simulink model "uav"  (R2024b)
settings: Solver=VariableStepAuto  StartTime=0.0  StopTime=30  RelTol=1e-3
libraries: slpidlib x3, shared6dof x1, aerolibadyn x1, aerolibanimutils x1
settings Model: Creator=91964  LastModifiedBy=91964

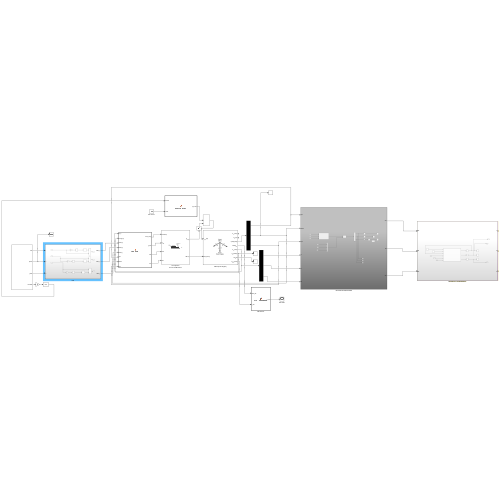
[thumbnail: Simulink's stored preview of the top-level diagram]
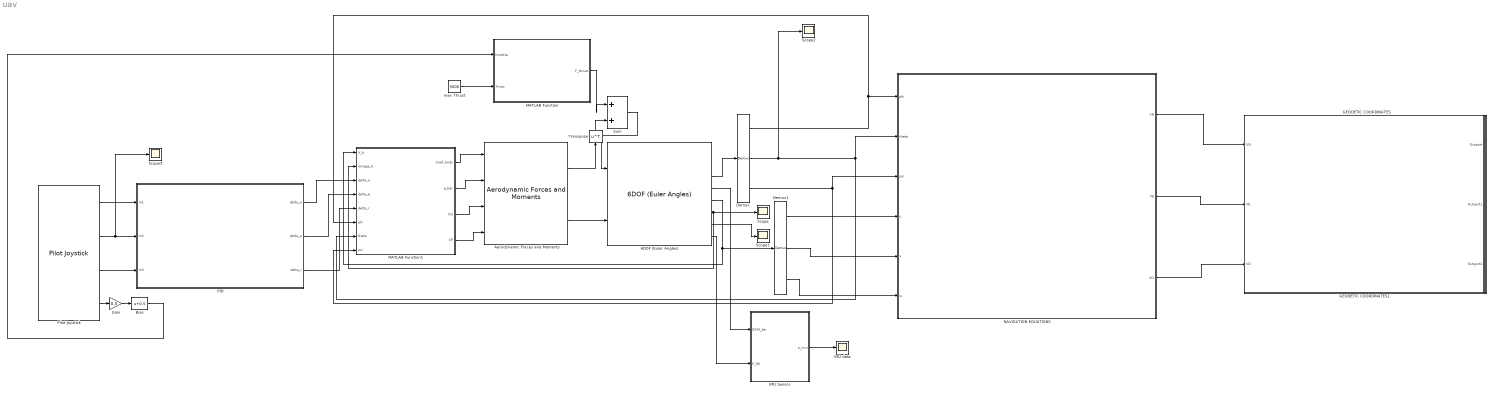
== system uav ==
  6DOF (Euler Angles) : shared6dof/6DOF (Euler Angles)  units=Metric (MKS)  mtype=Fixed  rep=Euler Angles  xme_0=[0 0 100]  Vm_0=[30 0 0]  eul_0=[0 0 0]  pm_0=[0 0 0]  mass_0=60  mass_e=0.5  mass_f=2.0  inertia=eye(3)  inertia_e=eye(3)  inertia_f=2*eye(3)  k_quat=1.0  vre_flag=on  abi_flag=off  aMode=0  xme_statename=''  Vm_statename=''  eul_statename=''  quat_statename=''  pm_statename=''  mass_statename=''
  "Aerodynamic Forces and Moments " : aerolibadyn/Aerodynamic Forces and Moments   inputAxes=Body  outputForceAxes=Body  outputMomentAxes=Body  S=1  b=1  cbar=1
  Bias : Bias  Bias=0.5  SaturateOnIntegerOverflow=off
  Demux : Demux  Outputs=3
  Demux1 : Demux  Outputs=3
  GEODETIC COORDINATES : Subsystem
  GEODETIC COORDINATES1 : Subsystem
  Gain : Gain  Gain=0.5
  IMU Sensor : MATLAB Function  TreatAsAtomicUnit=on
  IMU data : Scope
  MATLAB Function : MATLAB Function  TreatAsAtomicUnit=on
  MATLAB Function1 : MATLAB Function  TreatAsAtomicUnit=on
  NAVIGATION EQUATIONS : Subsystem
  PID : Subsystem
  Pilot Joystick : aerolibanimutils/Pilot Joystick  JoystickID=Joystick1  OutputConfiguration=FourAxis  SampleTime=1/30
  Scope{,1..3} (4 alike) : Scope
  Sum : Sum  Inputs=|++
  Transpose : Math  Operator=transpose
  "max Thrust " : Constant  Value=5000
  wires:
  "Aerodynamic Forces and Moments "/1 -> Transpose/1
  "Aerodynamic Forces and Moments "/2 -> 6DOF (Euler Angles)/2
  NAVIGATION EQUATIONS/2(VE) -> GEODETIC COORDINATES/2(VE)
  NAVIGATION EQUATIONS/1(VN) -> GEODETIC COORDINATES/1(VN)
  NAVIGATION EQUATIONS/3(VD) -> GEODETIC COORDINATES/3(VD)
  Demux/2 -> MATLAB Function1/7(theta), NAVIGATION EQUATIONS/2(theta), Scope2/1
  6DOF (Euler Angles)/3 -> Demux/1
  Demux/3 -> MATLAB Function1/8(psi), NAVIGATION EQUATIONS/3(psi)
  6DOF (Euler Angles)/5 -> MATLAB Function1/1(V_b), Demux1/1
  Demux1/1 -> NAVIGATION EQUATIONS/4(u)
  Demux1/2 -> NAVIGATION EQUATIONS/5(v)
  Demux1/3 -> NAVIGATION EQUATIONS/6(w)
  Pilot Joystick/1 -> PID/1(In1)
  Pilot Joystick/2 -> Scope3/1, PID/2(In2)
  Pilot Joystick/3 -> PID/3(In3)
  PID/1(delta_a) -> MATLAB Function1/3(delta_a)
  PID/2(delta_e) -> MATLAB Function1/4(delta_e)
  PID/3(delta_r) -> MATLAB Function1/5(delta_r)
  6DOF (Euler Angles)/4 -> IMU Sensor/1(DCM_be)
  6DOF (Euler Angles)/8 -> IMU Sensor/2(A_bb)
  IMU Sensor/1(a_imu) -> IMU data/1
  6DOF (Euler Angles)/6 -> MATLAB Function1/2(omega_b), Scope/1
  6DOF (Euler Angles)/7 -> Scope1/1
  Pilot Joystick/4 -> Gain/1
  "max Thrust "/1 -> MATLAB Function/2(Tmax)
  Gain/1 -> Bias/1
  Bias/1 -> MATLAB Function/1(throttle)
  MATLAB Function/1(F_thrust) -> Sum/1
  Sum/1 -> 6DOF (Euler Angles)/1
  Transpose/1 -> Sum/2
  Demux/1 -> MATLAB Function1/6(phi), NAVIGATION EQUATIONS/1(phi)
  MATLAB Function1/1(Coef_body) -> "Aerodynamic Forces and Moments "/1
  MATLAB Function1/2(q_bar) -> "Aerodynamic Forces and Moments "/2
  MATLAB Function1/3(CG) -> "Aerodynamic Forces and Moments "/3
  MATLAB Function1/4(CP) -> "Aerodynamic Forces and Moments "/4

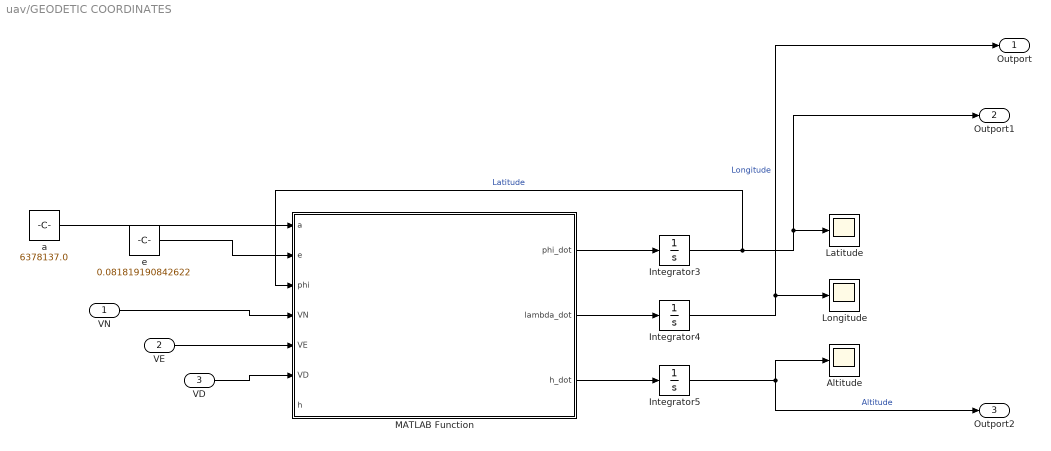
== system uav/GEODETIC COORDINATES ==
  VN : Inport
  VE : Inport  Port=2
  VD : Inport  Port=3
  Altitude : Scope
  Integrator3 : Integrator
  Integrator4 : Integrator
  Integrator5 : Integrator
  Latitude : Scope
  Longitude : Scope
  MATLAB Function : MATLAB Function  TreatAsAtomicUnit=on
  a : Constant  Value=6378137.0
  e : Constant  Value=0.081819190842622
  Outport : Outport
  Outport1 : Outport  Port=2
  Outport2 : Outport  Port=3
  wires:
  MATLAB Function/3(h_dot) -> Integrator5/1
  e/1 -> MATLAB Function/2(e)
  MATLAB Function/2(lambda_dot) -> Integrator4/1
  MATLAB Function/1(phi_dot) -> Integrator3/1
  a/1 -> MATLAB Function/1(a)
  Integrator4/1 -> Outport/1, Longitude/1  "Longitude"
  Integrator3/1 -> MATLAB Function/3(phi), Outport1/1, Latitude/1  "Latitude"
  Integrator5/1 -> Altitude/1, Outport2/1  "Altitude"
  VN/1 -> MATLAB Function/4(VN)
  VD/1 -> MATLAB Function/6(VD)
  VE/1 -> MATLAB Function/5(VE)

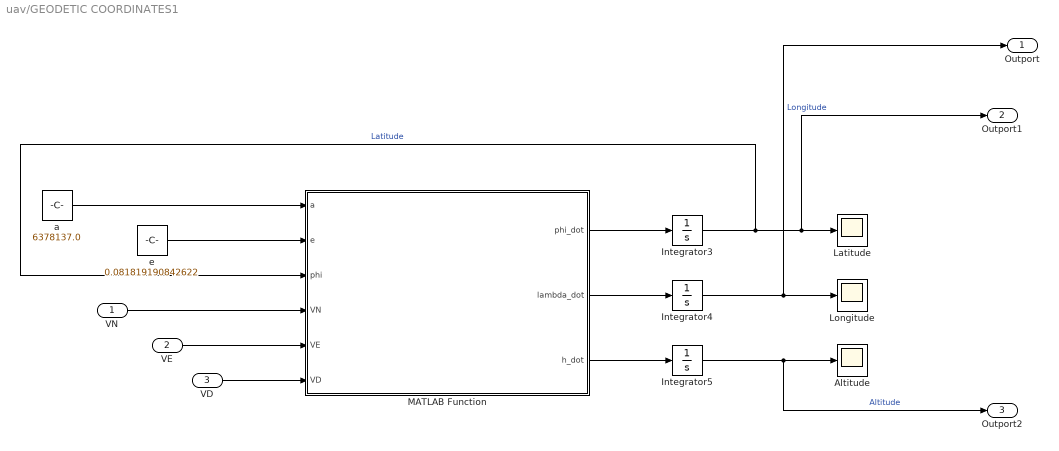
== system uav/GEODETIC COORDINATES1 ==
  VN : Inport
  VE : Inport  Port=2
  VD : Inport  Port=3
  Altitude : Scope
  Integrator3 : Integrator
  Integrator4 : Integrator
  Integrator5 : Integrator
  Latitude : Scope
  Longitude : Scope
  MATLAB Function : MATLAB Function  TreatAsAtomicUnit=on
  a : Constant  Value=6378137.0
  e : Constant  Value=0.081819190842622
  Outport : Outport
  Outport1 : Outport  Port=2
  Outport2 : Outport  Port=3
  wires:
  VE/1 -> MATLAB Function/5(VE)
  VD/1 -> MATLAB Function/6(VD)
  VN/1 -> MATLAB Function/4(VN)
  Integrator5/1 -> Altitude/1, Outport2/1  "Altitude"
  Integrator3/1 -> Latitude/1, Outport1/1, MATLAB Function/3(phi)  "Latitude"
  Integrator4/1 -> Longitude/1, Outport/1  "Longitude"
  a/1 -> MATLAB Function/1(a)
  MATLAB Function/1(phi_dot) -> Integrator3/1
  MATLAB Function/2(lambda_dot) -> Integrator4/1
  e/1 -> MATLAB Function/2(e)
  MATLAB Function/3(h_dot) -> Integrator5/1

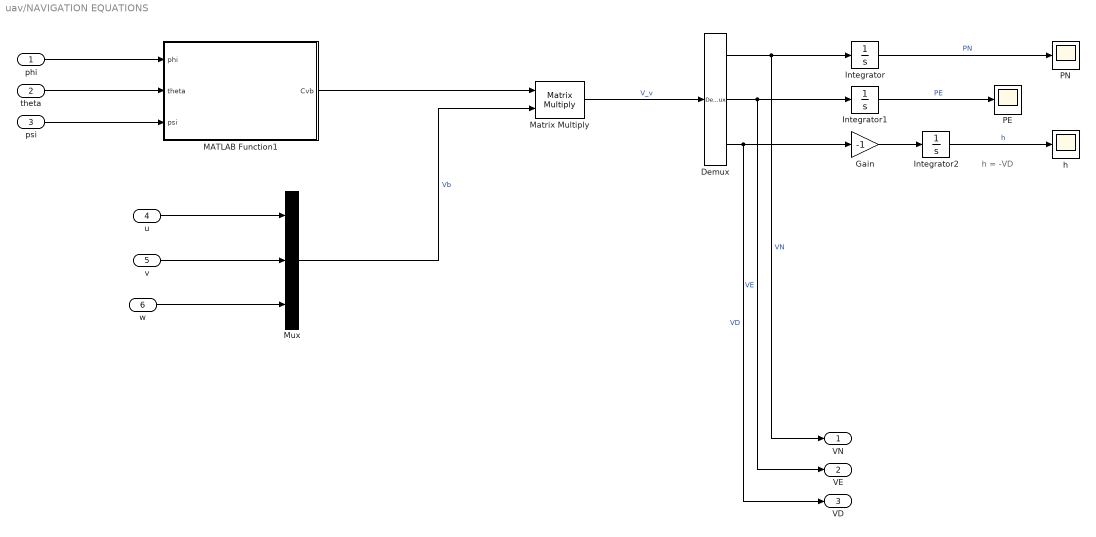
== system uav/NAVIGATION EQUATIONS ==
  note: h = -VD
  phi : Inport
  theta : Inport  Port=2
  psi : Inport  Port=3
  u : Inport  Port=4
  v : Inport  Port=5
  w : Inport  Port=6
  Demux : Demux  Outputs=3
  Gain : Gain  Gain=-1
  Integrator : Integrator
  Integrator1 : Integrator
  Integrator2 : Integrator
  MATLAB Function1 : MATLAB Function  TreatAsAtomicUnit=on
  Matrix Multiply : Product  Multiplication=Matrix(*)
  Mux : Mux  Inputs=3
  PE : Scope
  PN : Scope
  h : Scope
  VN : Outport
  VE : Outport  Port=2
  VD : Outport  Port=3
  wires:
  Demux/1 -> VN/1, Integrator/1  "VN"
  Gain/1 -> Integrator2/1
  Demux/2 -> VE/1, Integrator1/1  "VE"
  Mux/1 -> Matrix Multiply/2  "Vb"
  MATLAB Function1/1(Cvb) -> Matrix Multiply/1
  Demux/3 -> VD/1, Gain/1  "VD"
  v/1 -> Mux/2
  Integrator/1 -> PN/1  "PN"
  Matrix Multiply/1 -> Demux/1  "V_v"
  Integrator1/1 -> PE/1  "PE"
  Integrator2/1 -> h/1  "h"
  theta/1 -> MATLAB Function1/2(theta)
  psi/1 -> MATLAB Function1/3(psi)
  w/1 -> Mux/3
  u/1 -> Mux/1
  phi/1 -> MATLAB Function1/1(phi)

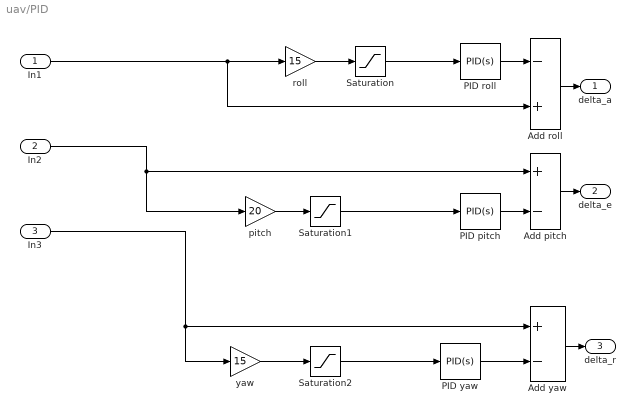
== system uav/PID ==
  In1 : Inport
  In2 : Inport  Port=2
  In3 : Inport  Port=3
  Add pitch : Sum  Inputs=+-
  Add roll : Sum  Inputs=-+
  Add yaw : Sum  Inputs=+-
  PID pitch : slpidlib/PID Controller  Controller=PID  Form=Parallel  TimeDomain=Continuous-time  UseExternalTs=off  SampleTime=-1  IntegratorMethod=Forward Euler  FilterMethod=Forward Euler  ControllerParametersSource=internal  P=1  I=1  UseKiTs=off  D=0  UseExternalDerivativeSource=off  N=100  UseFilter=on  TunerSelectOption=Transfer Function Based (PID Tuner App)  InitialConditionSource=internal  InitialConditionForIntegrator=0  InitialConditionForFilter=0  DifferentiatorICPrevScaledInput=0  ExternalReset=none  TrackingMode=off  Kt=1  LimitOutput=off  SatLimitsSource=internal  UpperSaturationLimit=inf  LowerSaturationLimit=-inf  LinearizeAsGain=on  AntiWindupMode=none  Kb=1  LimitIntegrator=off  UpperIntegratorSaturationLimit=inf  LowerIntegratorSaturationLimit=-inf  POutMin=[]  POutMax=[]  IOutMin=[]  IOutMax=[]  DOutMin=[]  DOutMax=[]  NOutMin=[]  NOutMax=[]  SumOutMin=[]  SumOutMax=[]  SaturationOutMin=[]  SaturationOutMax=[]  PParamMin=[]  PParamMax=[]  IParamMin=[]  IParamMax=[]  DParamMin=[]  DParamMax=[]  NParamMin=[]  NParamMax=[]  KbParamMin=[]  KbParamMax=[]  KtParamMin=[]  KtParamMax=[]  KbOutMin=[]  KbOutMax=[]  KtOutMin=[]  KtOutMax=[]  IntegratorOutMin=[]  IntegratorOutMax=[]  FilterOutMin=[]  FilterOutMax=[]  SumI1OutMin=[]  SumI1OutMax=[]  SumI2OutMin=[]  SumI2OutMax=[]  SumI3OutMin=[]  SumI3OutMax=[]  SumI4OutMin=[]  SumI4OutMax=[]  SumDOutMin=[]  SumDOutMax=[]  DifferentiatorOutMin=[]  DifferentiatorOutMax=[]  FilterDiffOutCoefMin=[]  FilterDiffOutCoefMax=[]  ReciprocalOutMin=[]  ReciprocalOutMax=[]  SumDenOutMin=[]  SumDenOutMax=[]  SumNumOutMin=[]  SumNumOutMax=[]  DivideOutMin=[]  DivideOutMax=[]  UdiffTsProdOutMin=[]  UdiffTsProdOutMax=[]  NTsProdOutMin=[]  NTsProdOutMax=[]  UintegralTsProdOutMin=[]  UintegralTsProdOutMax=[]  UngainTsProdOutMin=[]  UngainTsProdOutMax=[]  ClampingZeroOutDataTypeStr=Inherit: Inherit via back propagation  ClampingZeroOutMin=[]  ClampingZeroOutMax=[]  FilterDenConstantOutDataTypeStr=Inherit: Inherit via back propagation  FilterDenConstantOutMin=[]  FilterDenConstantOutMax=[]  PCopyOutDataTypeStr=Inherit: Inherit via back propagation  PCopyOutMin=[]  PCopyOutMax=[]  NCopyOutDataTypeStr=Inherit: Inherit via back propagation  NCopyOutMin=[]  NCopyOutMax=[]  IntegratorContinuousStateAttributes=''  IntegratorStateMustResolveToSignalObject=off  IntegratorRTWStateStorageClass=Auto  FilterContinuousStateAttributes=''  FilterStateMustResolveToSignalObject=off  FilterRTWStateStorageClass=Auto  ParallelPVariant=InternalParameters  IdealPVariant=Disabled  IVariant=InternalParameters  DVariant=InternalParameters  IntegratorVariant=Continuous  SatVariant=Disabled  AWVariant=Passthrough  PCopyVariant=Disabled  TRVariant=Disabled  FdbkBlocksVariant=Forward  IdealPFdbkVariant=Disabled  SatFdbkVariant=Disabled  DerivativeFilterVariant=ContFilter  NVariant=InternalParameters  NCopyVariant=Disabled  FilterICVariant=InternalICsFilter  IntegratorICVariant=InternalICs  ExternalResetVariant=Disabled  TRSumVariant=Passthrough  SumFdbkVariant=Disabled  SumVariant=Sum_PID  TsampFilterVariant=InternalTs  TsampNgainVariant=Passthrough  TsampIntegralVariant=Disabled_SignalSpec  ExternalSaturationOutDataTypeStr=Inherit: Same as second input  DerivativeSourceVariant=ErrorSignal  PreIntVariant=InternalPreInt
  PID roll : slpidlib/PID Controller  Controller=PID  Form=Parallel  TimeDomain=Continuous-time  UseExternalTs=off  SampleTime=-1  IntegratorMethod=Forward Euler  FilterMethod=Forward Euler  ControllerParametersSource=internal  P=1  I=1  UseKiTs=off  D=0  UseExternalDerivativeSource=off  N=100  UseFilter=on  TunerSelectOption=Transfer Function Based (PID Tuner App)  InitialConditionSource=internal  InitialConditionForIntegrator=0  InitialConditionForFilter=0  DifferentiatorICPrevScaledInput=0  ExternalReset=none  TrackingMode=off  Kt=1  LimitOutput=off  SatLimitsSource=internal  UpperSaturationLimit=inf  LowerSaturationLimit=-inf  LinearizeAsGain=on  AntiWindupMode=none  Kb=1  LimitIntegrator=off  UpperIntegratorSaturationLimit=inf  LowerIntegratorSaturationLimit=-inf  POutMin=[]  POutMax=[]  IOutMin=[]  IOutMax=[]  DOutMin=[]  DOutMax=[]  NOutMin=[]  NOutMax=[]  SumOutMin=[]  SumOutMax=[]  SaturationOutMin=[]  SaturationOutMax=[]  PParamMin=[]  PParamMax=[]  IParamMin=[]  IParamMax=[]  DParamMin=[]  DParamMax=[]  NParamMin=[]  NParamMax=[]  KbParamMin=[]  KbParamMax=[]  KtParamMin=[]  KtParamMax=[]  KbOutMin=[]  KbOutMax=[]  KtOutMin=[]  KtOutMax=[]  IntegratorOutMin=[]  IntegratorOutMax=[]  FilterOutMin=[]  FilterOutMax=[]  SumI1OutMin=[]  SumI1OutMax=[]  SumI2OutMin=[]  SumI2OutMax=[]  SumI3OutMin=[]  SumI3OutMax=[]  SumI4OutMin=[]  SumI4OutMax=[]  SumDOutMin=[]  SumDOutMax=[]  DifferentiatorOutMin=[]  DifferentiatorOutMax=[]  FilterDiffOutCoefMin=[]  FilterDiffOutCoefMax=[]  ReciprocalOutMin=[]  ReciprocalOutMax=[]  SumDenOutMin=[]  SumDenOutMax=[]  SumNumOutMin=[]  SumNumOutMax=[]  DivideOutMin=[]  DivideOutMax=[]  UdiffTsProdOutMin=[]  UdiffTsProdOutMax=[]  NTsProdOutMin=[]  NTsProdOutMax=[]  UintegralTsProdOutMin=[]  UintegralTsProdOutMax=[]  UngainTsProdOutMin=[]  UngainTsProdOutMax=[]  ClampingZeroOutDataTypeStr=Inherit: Inherit via back propagation  ClampingZeroOutMin=[]  ClampingZeroOutMax=[]  FilterDenConstantOutDataTypeStr=Inherit: Inherit via back propagation  FilterDenConstantOutMin=[]  FilterDenConstantOutMax=[]  PCopyOutDataTypeStr=Inherit: Inherit via back propagation  PCopyOutMin=[]  PCopyOutMax=[]  NCopyOutDataTypeStr=Inherit: Inherit via back propagation  NCopyOutMin=[]  NCopyOutMax=[]  IntegratorContinuousStateAttributes=''  IntegratorStateMustResolveToSignalObject=off  IntegratorRTWStateStorageClass=Auto  FilterContinuousStateAttributes=''  FilterStateMustResolveToSignalObject=off  FilterRTWStateStorageClass=Auto  ParallelPVariant=InternalParameters  IdealPVariant=Disabled  IVariant=InternalParameters  DVariant=InternalParameters  IntegratorVariant=Continuous  SatVariant=Disabled  AWVariant=Passthrough  PCopyVariant=Disabled  TRVariant=Disabled  FdbkBlocksVariant=Forward  IdealPFdbkVariant=Disabled  SatFdbkVariant=Disabled  DerivativeFilterVariant=ContFilter  NVariant=InternalParameters  NCopyVariant=Disabled  FilterICVariant=InternalICsFilter  IntegratorICVariant=InternalICs  ExternalResetVariant=Disabled  TRSumVariant=Passthrough  SumFdbkVariant=Disabled  SumVariant=Sum_PID  TsampFilterVariant=InternalTs  TsampNgainVariant=Passthrough  TsampIntegralVariant=Disabled_SignalSpec  ExternalSaturationOutDataTypeStr=Inherit: Same as second input  DerivativeSourceVariant=ErrorSignal  PreIntVariant=InternalPreInt
  PID yaw : slpidlib/PID Controller  Controller=PID  Form=Parallel  TimeDomain=Continuous-time  UseExternalTs=off  SampleTime=-1  IntegratorMethod=Forward Euler  FilterMethod=Forward Euler  ControllerParametersSource=internal  P=1  I=1  UseKiTs=off  D=0  UseExternalDerivativeSource=off  N=100  UseFilter=on  TunerSelectOption=Transfer Function Based (PID Tuner App)  InitialConditionSource=internal  InitialConditionForIntegrator=0  InitialConditionForFilter=0  DifferentiatorICPrevScaledInput=0  ExternalReset=none  TrackingMode=off  Kt=1  LimitOutput=off  SatLimitsSource=internal  UpperSaturationLimit=inf  LowerSaturationLimit=-inf  LinearizeAsGain=on  AntiWindupMode=none  Kb=1  LimitIntegrator=off  UpperIntegratorSaturationLimit=inf  LowerIntegratorSaturationLimit=-inf  POutMin=[]  POutMax=[]  IOutMin=[]  IOutMax=[]  DOutMin=[]  DOutMax=[]  NOutMin=[]  NOutMax=[]  SumOutMin=[]  SumOutMax=[]  SaturationOutMin=[]  SaturationOutMax=[]  PParamMin=[]  PParamMax=[]  IParamMin=[]  IParamMax=[]  DParamMin=[]  DParamMax=[]  NParamMin=[]  NParamMax=[]  KbParamMin=[]  KbParamMax=[]  KtParamMin=[]  KtParamMax=[]  KbOutMin=[]  KbOutMax=[]  KtOutMin=[]  KtOutMax=[]  IntegratorOutMin=[]  IntegratorOutMax=[]  FilterOutMin=[]  FilterOutMax=[]  SumI1OutMin=[]  SumI1OutMax=[]  SumI2OutMin=[]  SumI2OutMax=[]  SumI3OutMin=[]  SumI3OutMax=[]  SumI4OutMin=[]  SumI4OutMax=[]  SumDOutMin=[]  SumDOutMax=[]  DifferentiatorOutMin=[]  DifferentiatorOutMax=[]  FilterDiffOutCoefMin=[]  FilterDiffOutCoefMax=[]  ReciprocalOutMin=[]  ReciprocalOutMax=[]  SumDenOutMin=[]  SumDenOutMax=[]  SumNumOutMin=[]  SumNumOutMax=[]  DivideOutMin=[]  DivideOutMax=[]  UdiffTsProdOutMin=[]  UdiffTsProdOutMax=[]  NTsProdOutMin=[]  NTsProdOutMax=[]  UintegralTsProdOutMin=[]  UintegralTsProdOutMax=[]  UngainTsProdOutMin=[]  UngainTsProdOutMax=[]  ClampingZeroOutDataTypeStr=Inherit: Inherit via back propagation  ClampingZeroOutMin=[]  ClampingZeroOutMax=[]  FilterDenConstantOutDataTypeStr=Inherit: Inherit via back propagation  FilterDenConstantOutMin=[]  FilterDenConstantOutMax=[]  PCopyOutDataTypeStr=Inherit: Inherit via back propagation  PCopyOutMin=[]  PCopyOutMax=[]  NCopyOutDataTypeStr=Inherit: Inherit via back propagation  NCopyOutMin=[]  NCopyOutMax=[]  IntegratorContinuousStateAttributes=''  IntegratorStateMustResolveToSignalObject=off  IntegratorRTWStateStorageClass=Auto  FilterContinuousStateAttributes=''  FilterStateMustResolveToSignalObject=off  FilterRTWStateStorageClass=Auto  ParallelPVariant=InternalParameters  IdealPVariant=Disabled  IVariant=InternalParameters  DVariant=InternalParameters  IntegratorVariant=Continuous  SatVariant=Disabled  AWVariant=Passthrough  PCopyVariant=Disabled  TRVariant=Disabled  FdbkBlocksVariant=Forward  IdealPFdbkVariant=Disabled  SatFdbkVariant=Disabled  DerivativeFilterVariant=ContFilter  NVariant=InternalParameters  NCopyVariant=Disabled  FilterICVariant=InternalICsFilter  IntegratorICVariant=InternalICs  ExternalResetVariant=Disabled  TRSumVariant=Passthrough  SumFdbkVariant=Disabled  SumVariant=Sum_PID  TsampFilterVariant=InternalTs  TsampNgainVariant=Passthrough  TsampIntegralVariant=Disabled_SignalSpec  ExternalSaturationOutDataTypeStr=Inherit: Same as second input  DerivativeSourceVariant=ErrorSignal  PreIntVariant=InternalPreInt
  Saturation : Saturate  UpperLimit=15  LowerLimit=-15
  Saturation1 : Saturate  UpperLimit=20  LowerLimit=-20
  Saturation2 : Saturate  UpperLimit=15  LowerLimit=-15
  pitch : Gain  Gain=20
  roll : Gain  Gain=15
  yaw : Gain  Gain=15
  delta_a : Outport
  delta_e : Outport  Port=2
  delta_r : Outport  Port=3
  wires:
  pitch/1 -> Saturation1/1
  In2/1 -> Add pitch/1, pitch/1
  Add roll/1 -> delta_a/1
  In1/1 -> Add roll/2, roll/1
  Add yaw/1 -> delta_r/1
  PID pitch/1 -> Add pitch/2
  In3/1 -> Add yaw/1, yaw/1
  yaw/1 -> Saturation2/1
  PID roll/1 -> Add roll/1
  roll/1 -> Saturation/1
  Add pitch/1 -> delta_e/1
  PID yaw/1 -> Add yaw/2
  Saturation/1 -> PID roll/1
  Saturation1/1 -> PID pitch/1
  Saturation2/1 -> PID yaw/1

== matlab function uav/NAVIGATION EQUATIONS/MATLAB Function1 ==
  data: phi input; Cvb output; theta input; psi input
function Cvb = rotation_matrix_full(phi, theta, psi)
% This function computes the rotation matrices A*B, D*C, and their transpose F
% Inputs: phi, theta, psi (Euler angles in radians)
% Output: F (3x3 matrix, transpose of the full rotation matrix)
% Matrix C1v
C1v = [cos(psi), sin(psi), 0;
     -sin(psi), cos(psi), 0;
     0, 0, 1];

% Matrix C21
C21 = [cos(theta), 0, -sin(theta);
     0, 1, 0;
     sin(theta), 0, cos(theta)];

% Matrix Cb2
Cb2 = [1, 0, 0;
     0, cos(phi), sin(phi);
     0, -sin(phi), cos(phi)];
Cbv = Cb2*C21*C1v
Cvb = transpose(Cbv)

== matlab function uav/GEODETIC COORDINATES/MATLAB Function ==
  data: a input; phi_dot output; e input; phi input; VN input; VE input; VD input; lambda_dot output; h_dot output; h input
function [phi_dot, lambda_dot, h_dot] = wgs84_motion(a, e, phi, VN, VE, VD,h)
    % WGS-84 Motion Calculation
    % Inputs:
    % a  - Semi-major axis (meters)
    % e  - Eccentricity
    % phi - Latitude (radians)
    % h  - Altitude (meters)
    % VN - North velocity (m/s)
    % VE - East velocity (m/s)
    % VD - Down velocity (m/s)
    % Outputs:
    % phi_dot   - Latitude rate (rad/s)
    % lambda_dot - Longitude rate (rad/s)
    % h_dot     - Altitude rate (m/s)

    % Compute radius of curvature in the meridian (M)
    M = (a * (1 - e^2)) / (1 - e^2 * sin(phi)^2)^(3/2);
    
    % Compute radius of curvature in the prime vertical (N)
    N = a / sqrt(1 - e^2 * sin(phi)^2);
    
    % Compute latitude rate (phi_dot)
    phi_dot = VN / (M + h);
    
    % Compute longitude rate (lambda_dot)
    lambda_dot = VE / ((N + h) * cos(phi));
    
    % Compute altitude rate (h_dot)
    h_dot = -VD;
end

== matlab function uav/IMU Sensor ==
  settings: updateMethod=DISCRETE
  data: DCM_be input; A_bb input; a_imu output
function a_imu = IMU_Accelerometer(DCM_be, A_bb)
% Simulates accelerometer readings in the Earth frame (IMU output)
%
% Inputs:
%   A_bb    - Body acceleration vector [ax; ay; az] (m/s²)
%   DCM_be  - Direction Cosine Matrix (DCM) from body to Earth
%
% Output:
%   a_imu - Simulated IMU accelerometer readings in Earth frame

    % Define Earth's gravity in the Earth frame
    g_earth = [0; 0; -9.81]; % Gravity in m/s²
    
    % Convert Body Acceleration to Earth Frame
    A_earth = DCM_be * A_bb; 
    
    % Add Gravity Effect (IMU measures acceleration + gravity)
    a_imu = A_earth + g_earth;  
    
    % Add Sensor Bias (constant offset)
    bias = [0.02; -0.03; 0.01]; % Example bias in m/s²
    a_imu = a_imu + bias;
    
    % Add Sensor Noise (Gaussian noise to simulate sensor imperfections)
    noise_std_dev = [0.05; 0.05; 0.05]; % Standard deviation for noise
    noise = noise_std_dev .* randn(3,1);
    a_imu = a_imu + noise;
end

== matlab function uav/MATLAB Function ==
  data: throttle input; F_thrust output; Tmax input
function F_thrust = propulsion_system(throttle, Tmax)
% PROPULSION_SYSTEM Converts throttle input into thrust force
%
% Inputs:
%   throttle - Throttle input (0 to 1)
%   Tmax     - Maximum thrust (N)
%
% Output:
%   F_thrust - Thrust force vector in body frame [Fx; Fy; Fz]

% Ensure throttle is within bounds (0 to 1)
throttle = max(0, min(1, throttle));

% Compute thrust force in X direction
Fx = throttle * Tmax;
Fy = 0;  % No lateral thrust
Fz = 0;  % No vertical thrust

% Output thrust force as a vector in body frame
F_thrust = [Fx; Fy; Fz];

end

== matlab function uav/GEODETIC COORDINATES1/MATLAB Function ==
  data: a input; phi_dot output; e input; phi input; VN input; VE input; VD input; lambda_dot output; h_dot output
function [phi_dot, lambda_dot, h_dot] = wgs84_motion(a, e, phi, VN, VE, VD)
    % WGS-84 Motion Calculation
    % Inputs:
    % a  - Semi-major axis (meters)
    % e  - Eccentricity
    % phi - Latitude (radians)
    % h  - Altitude (meters)
    % VN - North velocity (m/s)
    % VE - East velocity (m/s)
    % VD - Down velocity (m/s)
    % Outputs:
    % phi_dot   - Latitude rate (rad/s)
    % lambda_dot - Longitude rate (rad/s)
    % h_dot     - Altitude rate (m/s)

    % Compute radius of curvature in the meridian (M)
    M = (a * (1 - e^2)) / (1 - e^2 * sin(phi)^2)^(3/2);
    h = -VD;
    
    % Compute radius of curvature in the prime vertical (N)
    N = a / sqrt(1 - e^2 * sin(phi)^2);
    
    % Compute latitude rate (phi_dot)
    phi_dot = VN / (M + h);
    
    % Compute longitude rate (lambda_dot)
    lambda_dot = VE / ((N + h) * cos(phi));
    
    % Compute altitude rate (h_dot)
    h_dot = -VD;
end

== matlab function uav/MATLAB Function1 ==
  data: V_b input; Coef_body output; q_bar output; omega_b input; delta_a input; delta_e input; delta_r input; phi input; theta input; psi input; CG output; CP output
function [Coef_body, q_bar, CG, CP] = aero_inputs(V_b, omega_b, delta_a, delta_e, delta_r, phi, theta, psi)
    % Inputs:
    % V_b    -> Velocity in body frame [u, v, w] (m/s)
    % omega_b -> Angular rates in body frame [p, q, r] (rad/s)
    % phi, theta, psi -> Euler angles (rad)
    % delta_a -> Aileron deflection (deg)
    % delta_e -> Elevator deflection (deg)
    % delta_r -> Rudder deflection (deg)

    % Extract velocity components
    u = V_b(1); % Forward velocity
    v = V_b(2); % Side velocity
    w = V_b(3); % Downward velocity

    % Extract angular rates
    p = omega_b(1); % Roll rate
    q = omega_b(2); % Pitch rate
    r = omega_b(3); % Yaw rate

    % Compute airspeed magnitude
    V = sqrt(u^2 + v^2 + w^2);
    
    % Prevent division by zero
    if V < 1e-6
        V = 1e-6;
    end

    % Compute angle of attack (alpha) and sideslip (beta)
    alpha = atan2(w, u);  % Angle of attack (rad)
    beta = asin(v / V);   % Sideslip angle (rad)

    % Example aerodynamic coefficients (replace with actual data)
    CL_0 = 0.2;        % Zero-lift coefficient
    CL_alpha = 5.5;    % Lift curve slope per rad
    CD_0 = 0.02;       % Zero-lift drag coefficient
    CM_0 = 0;          % Pitching moment coefficient at zero AoA
    CM_alpha = -1.2;   % Pitching moment slope
    CM_q = -5.0;       % Pitch damping
    CY_beta = -0.98;   % Side force coefficient per rad
    Cl_beta = -0.12;   % Roll moment due to sideslip
    Cl_p = -0.26;      % Roll damping
    Cl_r = 0.14;       % Roll due to yaw rate
    Cm_delta_e = -1.2; % Pitching moment due to elevator
    Cn_beta = 0.25;    % Yaw moment due to sideslip
    Cn_p = -0.02;      % Yaw due to roll rate
    Cn_r = -0.2;       % Yaw damping
    Cn_delta_r = -0.10;% Yaw moment due to rudder

    % Air properties
    rho = 1.225;  % Air density (kg/m³)
    S = 1.5;      % Wing area (m²)
    c = 0.3;      % Mean aerodynamic chord (m)
    b = 1.2;      % Wingspan (m)

    % Compute dynamic pressure
    q_bar = 0.5 * rho * V^2; % Dynamic pressure (N/m²)

    % Influence of Euler angles on aerodynamic forces
    phi_effect = cos(phi); % Roll effect on lift
    theta_effect = cos(theta); % Pitch effect on drag
    psi_effect = sin(psi); % Yaw effect on side force

    % Compute aerodynamic coefficients with Euler angle influence
    CL = (CL_0 + CL_alpha * alpha + CM_q * (q * c / (2*V))) * phi_effect;
    CD = (CD_0 + 0.1 * CL^2) * theta_effect; % Approximate quadratic drag model
    CY = CY_beta * beta * psi_effect;

    Cl = (Cl_beta * beta + Cl_p * (p * b / (2*V)) + Cl_r * (r * b / (2*V)) + deg2rad(delta_a)) * phi_effect;
    Cm = (CM_0 + CM_alpha * alpha + Cm_delta_e * deg2rad(delta_e)) * theta_effect;
    Cn = (Cn_beta * beta + Cn_p * (p * b / (2*V)) + Cn_r * (r * b / (2*V)) + Cn_delta_r * deg2rad(delta_r)) * psi_effect;

    % Pack coefficients into a vector (forces: X, Y, Z, moments: L, M, N)
    Coef_body = [ -CD, CY, -CL, Cl, Cm, Cn ]; % Body-frame coefficients

    % Define CG and CP locations (example values, modify as needed)
    CG = [0.1, 0, 0];  % [x, y, z] position of CG in body frame (m)
    CP = [0.2, 0, -0.05]; % [x, y, z] position of CP in body frame (m)

end
